simulink model "gm_inc_enc_v25_vnl"  (R2022a)
settings: Solver=FixedStepDiscrete  StartTime=0.0  StopTime=SimulationsDauer  RelTol=1e-3
undefined symbols (not defined in the file or in its folder): DiscIntNeverNeededParam, f_ISR, IncPerTurn, inital_zero_speed_timeout, n_max, OmegaPerOverSampl, Periode, Phase_Delay_A, Phase_Delay_B, PolePair, QuadratureFactor, reciprocal_iterations, T_fpga, T_mech
libraries: simulink x19, hdlsllib x11, hdlmdlgenlib x4, dspsrcs4 x3, dspswit3 x2, spsEdgeDetectorLib x2, simulink_extras x1
(part 1 of 4)
settings Model: Creator=Wendel_ELSYS  LastModifiedBy=ga92wum
settings SolverCC: ConcurrentTasks=on  AlgebraicLoopSolver=TrustRegion  MinimalZcImpactIntegration=on
settings DataIOCC: LimitDataPoints=on  SaveFormat=Array
settings OptimizationCC: BlockReduction=off  ConditionallyExecuteInputs=off  DefaultParameterBehavior=Inlined  InheritOutputTypeSmallerThanSingle=on  LifeSpan=inf
settings DebuggingCC: ReadBeforeWriteMsg=DisableAll  WriteAfterWriteMsg=DisableAll  WriteAfterReadMsg=DisableAll  AlgebraicLoopMsg=error  InheritedTsInSrcMsg=none  SingleTaskRateTransMsg=error  ParameterOverflowMsg=none  UnconnectedInputMsg=warning  UnconnectedOutputMsg=warning  UnconnectedLineMsg=warning  SFUnexpectedBacktrackingDiag=warning  SFNoUnconditionalDefaultTransitionDiag=warning  SFExecutionAtInitializationDiag=none  SFMachineParentedDataDiag=warning  ArithmeticOperatorsInVariantConditions=warning
settings HardwareCC: ProdBitPerPointer=32  ProdBitPerSizeT=32  ProdBitPerPtrDiffT=32  ProdLargestAtomicFloat=None  ProdIntDivRoundTo=Undefined  ProdEndianess=Unspecified  ProdWordSize=32  ProdHWDeviceType=ASIC/FPGA->ASIC/FPGA  ProdEqTarget=off
settings ModelReferenceCC: UpdateModelReferenceTargets=IfOutOfDate  PropagateSignalLabelsOutOfModel=off
settings SFSimCC: SFSimEcho=off  SimUseLocalCustomCode=off  CustomCodeUndefinedFunction=UseInterfaceOnly
settings RTWCC: RTWUseLocalCustomCode=off  DLArmComputeVersion=19.05
settings CodeAppCC: StateflowObjectComments=on
settings GRTTargetCC: TargetLangStandard=C89/C90 (ANSI)
settings ConfigComp: CovMetricSettings=dw  CovSaveCumulativeToWorkspaceVar=on  CovSaveSingleToWorkspaceVar=on  CovExternalEMLEnable=off

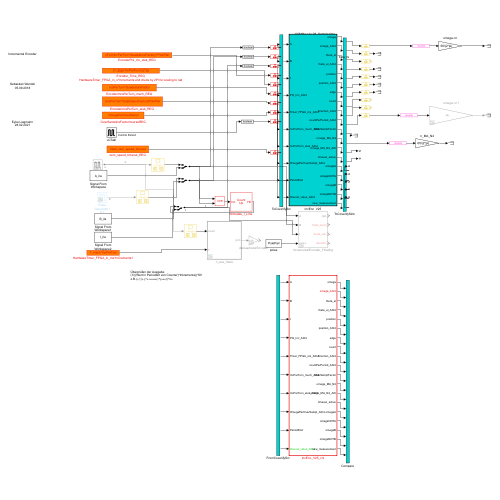
[thumbnail: Simulink's stored preview of the top-level diagram]
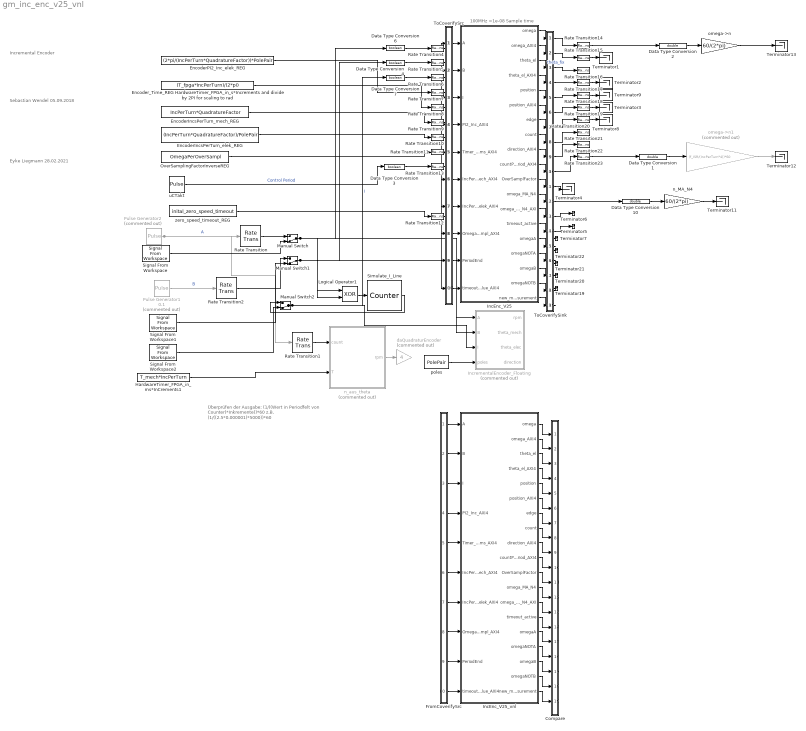
== system gm_inc_enc_v25_vnl ==
  note: 100MHz =1e-08 Sample time
  note: Überprüfen der Ausgabe:
      | (1/((Wert in Periodfelt von Counter)*Inkremente))*60
      | z.B. (1/((2.5*0.000001)*5000))*60
  note: Sebastian Wendel
      | 05.09.2018
  note: Incremental Encoder
  note: Eyke Liegmann
      | 28.02.2021
  Compare : Subsystem
      mask Display: disp('')
  Data Type Conversion1 : DataTypeConversion  OutDataTypeStr=double  SaturateOnIntegerOverflow=off  RndMeth=Floor
  Data Type Conversion10 : DataTypeConversion  OutDataTypeStr=double  SaturateOnIntegerOverflow=off  RndMeth=Floor
  Data Type Conversion2 : DataTypeConversion  OutDataTypeStr=double  SaturateOnIntegerOverflow=off  RndMeth=Floor
  Data Type Conversion{3..4,6..7} (4 alike) : DataTypeConversion  OutDataTypeStr=boolean  SaturateOnIntegerOverflow=off  RndMeth=Floor
  "EncoderIncsPerTurn_elek_REG " : Constant  Value=(IncPerTurn*QuadratureFactor)/PolePair  OutDataTypeStr=fixdt(0,16,0)  SampleTime=T_mech
  EncoderIncsPerTurn_mech_REG : Constant  Value=IncPerTurn*QuadratureFactor  OutDataTypeStr=fixdt(0,16,0)  SampleTime=T_mech
  EncoderPI2_Inc_elek_REG : Constant  Value=(2*pi/(IncPerTurn*QuadratureFactor))*PolePair  OutDataTypeStr=fixdt(0,24,24)  SampleTime=T_mech
  Encoder_Time_REG HardwareTimer_FPGA_in_s*Increments and divide by 2PI for scaling to rad : Constant  Value=(T_fpga*IncPerTurn)/(2*pi)  OutDataTypeStr=fixdt(0,32,32)  SampleTime=T_mech
  FromCoverifySrc : Subsystem
      mask Display: disp('')
  HardwareTimer_FPGA_in_ms*InCrements1 : Constant  Value=T_mech*IncPerTurn  OutDataTypeStr=double  SampleTime=T_mech
  IncEnc_V25 : Subsystem  TreatAsAtomicUnit=on
  IncEnc_V25_vnl : Subsystem  TreatAsAtomicUnit=on
  IncrementalEncoder_Floating : Subsystem  Commented=on
  Logical Operator1 : Logic  Operator=XOR  AllPortsSameDT=off  OutDataTypeStr=boolean
  Manual Switch : ManualSwitch  CurrentSetting=0
  Manual Switch1 : ManualSwitch  CurrentSetting=0
  Manual Switch2 : ManualSwitch  CurrentSetting=0
  OverSamplingFactorInverseREG : Constant  Value=OmegaPerOverSampl  OutDataTypeStr=fixdt(1,24,11)  SampleTime=T_mech
  Pulse Generator1 0.1 : DiscretePulseGenerator  Commented=on  PulseType=Time based  Period=Periode  PulseWidth=50  PhaseDelay=Phase_Delay_B  SampleTime=T_mech  VectorParams1D=off
  Pulse Generator2 : DiscretePulseGenerator  Commented=on  PulseType=Time based  Period=Periode  PulseWidth=50  PhaseDelay=Phase_Delay_A  SampleTime=T_mech  VectorParams1D=off
  Rate Transition{,1..2,14..23} (13 alike) : RateTransition  Deterministic=off  OutPortSampleTime=T_mech
  Rate Transition{4..13} (10 alike) : RateTransition  Deterministic=off  OutPortSampleTime=T_fpga
  Signal From Workspace : dspsrcs4/Signal From Workspace  X=A_ila  Ts=T_mech  nsamps=1  OutputAfterFinalValue=Setting to zero  ignoreOrWarnInputAndFrameLengths=off  OutputFrames=off
  Signal From Workspace1 : dspsrcs4/Signal From Workspace  X=B_ila  Ts=T_mech  nsamps=1  OutputAfterFinalValue=Setting to zero  ignoreOrWarnInputAndFrameLengths=off  OutputFrames=off
  Signal From Workspace2 : dspsrcs4/Signal From Workspace  X=I_ila  Ts=T_mech  nsamps=1  OutputAfterFinalValue=Setting to zero  ignoreOrWarnInputAndFrameLengths=off  OutputFrames=off
  Simulate_I_Line : dspswit3/Counter  Direction=Up  CountEvent=Either edge  CounterSize=User defined  MaxCount=IncPerTurn*4  InitialCount=0  Output=Hit  HitValue=IncPerTurn*4  ResetInput=off  SamplesPerFrame=1  Ts=1  CntDtype=double  HitDtype=Boolean
  Terminator{1..9,11..13,19..22} (16 alike) : Terminator
  ToCoverifySink : Subsystem
      mask Display: disp('')
  ToCoverifySrc : Subsystem
      mask Display: disp('')
  "daQuadraturEncoder " : Gain  Commented=on  Gain=4
  n_MA_N4 : Gain  Gain=60/(2*pi)  OutDataTypeStr=double
  n_aus_theta : Subsystem  Commented=on  TreatAsAtomicUnit=on
  omega->n : Gain  Gain=60/(2*pi)  OutDataTypeStr=double
  omega->n1 : Gain  Commented=on  Gain=(f_ISR/(IncPerTurn*4))*60  OutDataTypeStr=double
  poles : Constant  Value=PolePair  OutDataTypeStr=uint8  SampleTime=T_mech
  uCTakt : DiscretePulseGenerator  PulseType=Time based  Period=1/f_ISR  PulseWidth=f_ISR*T_fpga *100  SampleTime=T_mech  VectorParams1D=off
  zero_speed_timeout_REG : Constant  Value=inital_zero_speed_timeout  OutDataTypeStr=uint32  SampleTime=T_mech
  wires:
  Pulse Generator1 0.1/1 -> Rate Transition2/1  "B"
  Manual Switch1/1 -> Logical Operator1/2, Data Type Conversion4/1, IncrementalEncoder_Floating/2(B)
  Manual Switch2/1 -> Data Type Conversion7/1, IncrementalEncoder_Floating/3(I)  "I"
  Logical Operator1/1 -> Simulate_I_Line/1
  Manual Switch/1 -> Data Type Conversion6/1, IncrementalEncoder_Floating/1(A), Logical Operator1/1
  Data Type Conversion6/1 -> Rate Transition4/1
  Data Type Conversion4/1 -> Rate Transition5/1
  Data Type Conversion7/1 -> Rate Transition6/1
  poles/1 -> IncrementalEncoder_Floating/4(poles)
  EncoderPI2_Inc_elek_REG/1 -> Rate Transition7/1
  Encoder_Time_REG HardwareTimer_FPGA_in_s*Increments and divide by 2PI for scaling to rad/1 -> Rate Transition8/1
  EncoderIncsPerTurn_mech_REG/1 -> Rate Transition9/1
  "EncoderIncsPerTurn_elek_REG "/1 -> Rate Transition10/1
  omega->n/1 -> Terminator13/1
  Data Type Conversion2/1 -> omega->n/1
  HardwareTimer_FPGA_in_ms*InCrements1/1 -> n_aus_theta/2(T)
  Rate Transition1/1 -> n_aus_theta/1(count)
  n_aus_theta/1(rpm) -> "daQuadraturEncoder "/1
  Pulse Generator2/1 -> Rate Transition/1, Rate Transition1/1  "A"
  OverSamplingFactorInverseREG/1 -> Rate Transition11/1
  Rate Transition2/1 -> Manual Switch1/1
  Rate Transition/1 -> Manual Switch/1
  uCTakt/1 -> Data Type Conversion3/1  "Control Period"
  Data Type Conversion1/1 -> omega->n1/1
  Data Type Conversion3/1 -> Rate Transition13/1
  Rate Transition14/1 -> Data Type Conversion2/1
  Rate Transition15/1 -> Terminator1/1
  Rate Transition17/1 -> Terminator2/1
  Rate Transition19/1 -> Terminator3/1
  Rate Transition23/1 -> Data Type Conversion1/1
  Signal From Workspace/1 -> Manual Switch/2
  Signal From Workspace1/1 -> Manual Switch1/2
  Signal From Workspace2/1 -> Manual Switch2/2
  Simulate_I_Line/1 -> Manual Switch2/1
  Data Type Conversion10/1 -> n_MA_N4/1
  zero_speed_timeout_REG/1 -> Rate Transition12/1
  Rate Transition20/1 -> Terminator8/1
  Rate Transition18/1 -> Terminator9/1
  n_MA_N4/1 -> Terminator11/1
  omega->n1/1 -> Terminator12/1
  ToCoverifySrc/1(out1) -> IncEnc_V25/1(A)
  ToCoverifySrc/2(out2) -> IncEnc_V25/2(B)
  ToCoverifySrc/3(out3) -> IncEnc_V25/3(I)
  ToCoverifySrc/4(out4) -> IncEnc_V25/4(PI2_Inc_AXI4)
  ToCoverifySrc/5(out5) -> IncEnc_V25/5(Timer_FPGA_ms_AXI4)
  ToCoverifySrc/6(out6) -> IncEnc_V25/6(IncPerTurn_mech_AXI4)
  ToCoverifySrc/7(out7) -> IncEnc_V25/7(IncPerTurn_elek_AXI4)
  ToCoverifySrc/8(out8) -> IncEnc_V25/8(OmegaPerOverSampl_AXI4)
  ToCoverifySrc/9(out9) -> IncEnc_V25/9(PeriodEnd)
  ToCoverifySrc/10(out10) -> IncEnc_V25/10(timeout_value_AXI4)
  IncEnc_V25/1(omega) -> ToCoverifySink/1(in1)
  IncEnc_V25/2(omega_AXI4) -> ToCoverifySink/2(in2)
  IncEnc_V25/3(theta_el) -> ToCoverifySink/3(in3)  "theta_fix"
  IncEnc_V25/4(theta_el_AXI4) -> ToCoverifySink/4(in4)
  IncEnc_V25/5(position) -> ToCoverifySink/5(in5)
  IncEnc_V25/6(position_AXI4) -> ToCoverifySink/6(in6)
  IncEnc_V25/7(edge) -> ToCoverifySink/7(in7)
  IncEnc_V25/8(count) -> ToCoverifySink/8(in8)
  IncEnc_V25/9(direction_AXI4) -> ToCoverifySink/9(in9)
  IncEnc_V25/10(countPerPeriod_AXI4) -> ToCoverifySink/10(in10)
  IncEnc_V25/11(OverSamplFactor) -> ToCoverifySink/11(in11)
  IncEnc_V25/12(omega_MA_N4) -> ToCoverifySink/12(in12)
  IncEnc_V25/13(omega_MA_N4_AXI) -> ToCoverifySink/13(in13)
  IncEnc_V25/14(timeout_active) -> ToCoverifySink/14(in14)
  IncEnc_V25/15(omegaA) -> ToCoverifySink/15(in15)
  IncEnc_V25/16(omegaNOTA) -> ToCoverifySink/16(in16)
  IncEnc_V25/17(omegaB) -> ToCoverifySink/17(in17)
  IncEnc_V25/18(omegaNOTB) -> ToCoverifySink/18(in18)
  IncEnc_V25/19(new_measurement) -> ToCoverifySink/19(in19)
  Rate Transition4/1 -> ToCoverifySrc/1(in1)
  Rate Transition5/1 -> ToCoverifySrc/2(in2)
  Rate Transition6/1 -> ToCoverifySrc/3(in3)
  Rate Transition7/1 -> ToCoverifySrc/4(in4)
  Rate Transition8/1 -> ToCoverifySrc/5(in5)
  Rate Transition9/1 -> ToCoverifySrc/6(in6)
  Rate Transition10/1 -> ToCoverifySrc/7(in7)
  Rate Transition11/1 -> ToCoverifySrc/8(in8)
  Rate Transition13/1 -> ToCoverifySrc/9(in9)
  Rate Transition12/1 -> ToCoverifySrc/10(in10)
  ToCoverifySink/1(out1) -> Rate Transition14/1
  ToCoverifySink/2(out2) -> Rate Transition15/1
  ToCoverifySink/3(out3) -> Rate Transition16/1
  ToCoverifySink/4(out4) -> Rate Transition17/1
  ToCoverifySink/5(out5) -> Rate Transition18/1
  ToCoverifySink/6(out6) -> Rate Transition19/1
  ToCoverifySink/7(out7) -> Rate Transition20/1
  ToCoverifySink/8(out8) -> Rate Transition21/1
  ToCoverifySink/9(out9) -> Rate Transition22/1
  ToCoverifySink/10(out10) -> Rate Transition23/1
  ToCoverifySink/11(out11) -> Terminator4/1
  ToCoverifySink/12(out12) -> Data Type Conversion10/1
  ToCoverifySink/13(out13) -> Terminator6/1
  ToCoverifySink/14(out14) -> Terminator5/1
  ToCoverifySink/15(out15) -> Terminator7/1
  ToCoverifySink/16(out16) -> Terminator22/1
  ToCoverifySink/17(out17) -> Terminator21/1
  ToCoverifySink/18(out18) -> Terminator20/1
  ToCoverifySink/19(out19) -> Terminator19/1
  FromCoverifySrc/1(out1) -> IncEnc_V25_vnl/1(A)
  FromCoverifySrc/2(out2) -> IncEnc_V25_vnl/2(B)
  FromCoverifySrc/3(out3) -> IncEnc_V25_vnl/3(I)
  FromCoverifySrc/4(out4) -> IncEnc_V25_vnl/4(PI2_Inc_AXI4)
  FromCoverifySrc/5(out5) -> IncEnc_V25_vnl/5(Timer_FPGA_ms_AXI4)
  FromCoverifySrc/6(out6) -> IncEnc_V25_vnl/6(IncPerTurn_mech_AXI4)
  FromCoverifySrc/7(out7) -> IncEnc_V25_vnl/7(IncPerTurn_elek_AXI4)
  FromCoverifySrc/8(out8) -> IncEnc_V25_vnl/8(OmegaPerOverSampl_AXI4)
  FromCoverifySrc/9(out9) -> IncEnc_V25_vnl/9(PeriodEnd)
  FromCoverifySrc/10(out10) -> IncEnc_V25_vnl/10(timeout_value_AXI4)
  IncEnc_V25_vnl/1(omega) -> Compare/1(in1)
  IncEnc_V25_vnl/2(omega_AXI4) -> Compare/2(in2)
  IncEnc_V25_vnl/3(theta_el) -> Compare/3(in3)
  IncEnc_V25_vnl/4(theta_el_AXI4) -> Compare/4(in4)
  IncEnc_V25_vnl/5(position) -> Compare/5(in5)
  IncEnc_V25_vnl/6(position_AXI4) -> Compare/6(in6)
  IncEnc_V25_vnl/7(edge) -> Compare/7(in7)
  IncEnc_V25_vnl/8(count) -> Compare/8(in8)
  IncEnc_V25_vnl/9(direction_AXI4) -> Compare/9(in9)
  IncEnc_V25_vnl/10(countPerPeriod_AXI4) -> Compare/10(in10)
  IncEnc_V25_vnl/11(OverSamplFactor) -> Compare/11(in11)
  IncEnc_V25_vnl/12(omega_MA_N4) -> Compare/12(in12)
  IncEnc_V25_vnl/13(omega_MA_N4_AXI) -> Compare/13(in13)
  IncEnc_V25_vnl/14(timeout_active) -> Compare/14(in14)
  IncEnc_V25_vnl/15(omegaA) -> Compare/15(in15)
  IncEnc_V25_vnl/16(omegaNOTA) -> Compare/16(in16)
  IncEnc_V25_vnl/17(omegaB) -> Compare/17(in17)
  IncEnc_V25_vnl/18(omegaNOTB) -> Compare/18(in18)
  IncEnc_V25_vnl/19(new_measurement) -> Compare/19(in19)

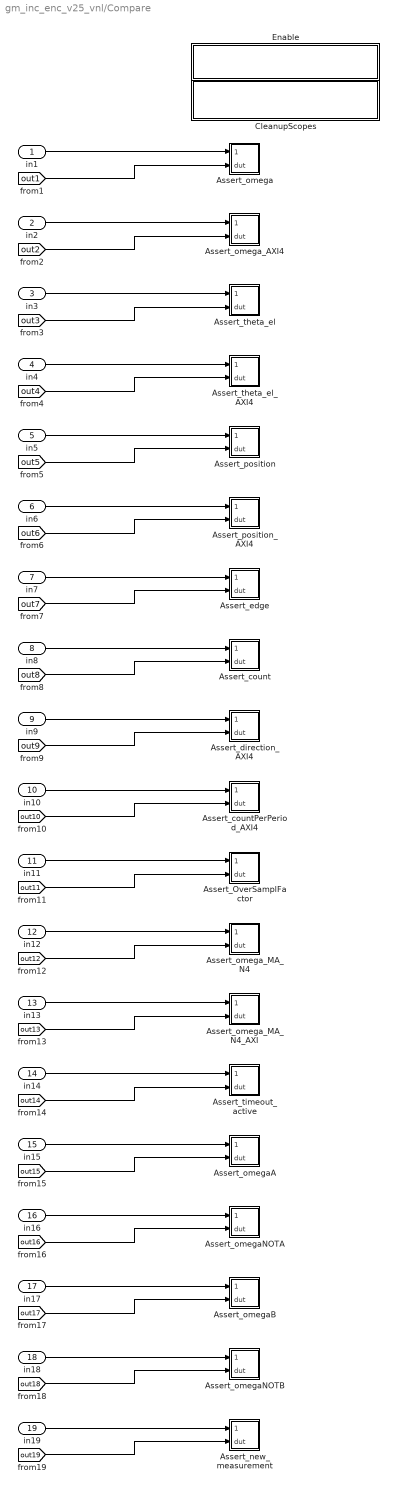
== system gm_inc_enc_v25_vnl/Compare ==
  in1 : Inport
  in2 : Inport  Port=2
  in3 : Inport  Port=3
  in4 : Inport  Port=4
  in5 : Inport  Port=5
  in6 : Inport  Port=6
  in7 : Inport  Port=7
  in8 : Inport  Port=8
  in9 : Inport  Port=9
  in10 : Inport  Port=10
  in11 : Inport  Port=11
  in12 : Inport  Port=12
  in13 : Inport  Port=13
  in14 : Inport  Port=14
  in15 : Inport  Port=15
  in16 : Inport  Port=16
  in17 : Inport  Port=17
  in18 : Inport  Port=18
  in19 : Inport  Port=19
  Assert_OverSamplFactor : Subsystem
  Assert_count : Subsystem
  Assert_countPerPeriod_AXI4 : Subsystem
  Assert_direction_AXI4 : Subsystem
  Assert_edge : Subsystem
  Assert_new_measurement : Subsystem
  Assert_omega : Subsystem
  Assert_omegaA : Subsystem
  Assert_omegaB : Subsystem
  Assert_omegaNOTA : Subsystem
  Assert_omegaNOTB : Subsystem
  Assert_omega_AXI4 : Subsystem
  Assert_omega_MA_N4 : Subsystem
  Assert_omega_MA_N4_AXI : Subsystem
  Assert_position : Subsystem
  Assert_position_AXI4 : Subsystem
  Assert_theta_el : Subsystem
  Assert_theta_el_AXI4 : Subsystem
  Assert_timeout_active : Subsystem
  CleanupScopes : Subsystem
      settings: OpenFcn=|
      | blkName = gcb; %self block
      | idx = regexp(blkName, '/CleanupScopes$', 'once');
      | blkParent = blkName(1:idx-1);
      | blks=find_system(blkParent, 'LookUnderMasks', 'all','blocktype', 'Scope');
      | for itr = 1:length(blks)
      | 	 hScopeCfg = get_param(blks{itr},'ScopeConfiguration');
      | 	 hScopeCfg.Visible = ~ hScopeCfg.Visible;
      | end
      | drawnow;
      mask Display: fprintf(message('hdlcoder:cosim:vnl_dblclick').getString());
  Enable : Subsystem
      settings: OpenFcn=|
      | blkName = gcb;
      | idx = regexp(blkName, '/Enable$', 'once');
      | blkParent = blkName(1:idx-1);
      | blks=find_system(blkParent, 'LookUnderMasks', 'all','blocktype', 'Assertion');
      | e = get_param(blks{1}, 'Enabled');
      | if strcmp(e, 'on'), f= 'off';, else, f = 'on';, end
      | for ii=1:length(blks), set_param(blks{ii}, 'Enabled', f);, end
      | set_param(gcb, 'MaskDisplay',['fprintf(message(''hdlcoder:cosim:vnl_dblclick_assertions'',','''',upper(e),'''',').getString())']);
      mask Display: fprintf(message('hdlcoder:cosim:vnl_dblclick_assertions','OFF').getString());
  wires:
  in1/1 -> Assert_omega/1(cosim)
  [out1] -> Assert_omega/2(dut)
  in2/1 -> Assert_omega_AXI4/1(cosim)
  [out2] -> Assert_omega_AXI4/2(dut)
  in3/1 -> Assert_theta_el/1(cosim)
  [out3] -> Assert_theta_el/2(dut)
  in4/1 -> Assert_theta_el_AXI4/1(cosim)
  [out4] -> Assert_theta_el_AXI4/2(dut)
  in5/1 -> Assert_position/1(cosim)
  [out5] -> Assert_position/2(dut)
  in6/1 -> Assert_position_AXI4/1(cosim)
  [out6] -> Assert_position_AXI4/2(dut)
  in7/1 -> Assert_edge/1(cosim)
  [out7] -> Assert_edge/2(dut)
  in8/1 -> Assert_count/1(cosim)
  [out8] -> Assert_count/2(dut)
  in9/1 -> Assert_direction_AXI4/1(cosim)
  [out9] -> Assert_direction_AXI4/2(dut)
  in10/1 -> Assert_countPerPeriod_AXI4/1(cosim)
  [out10] -> Assert_countPerPeriod_AXI4/2(dut)
  in11/1 -> Assert_OverSamplFactor/1(cosim)
  [out11] -> Assert_OverSamplFactor/2(dut)
  in12/1 -> Assert_omega_MA_N4/1(cosim)
  [out12] -> Assert_omega_MA_N4/2(dut)
  in13/1 -> Assert_omega_MA_N4_AXI/1(cosim)
  [out13] -> Assert_omega_MA_N4_AXI/2(dut)
  in14/1 -> Assert_timeout_active/1(cosim)
  [out14] -> Assert_timeout_active/2(dut)
  in15/1 -> Assert_omegaA/1(cosim)
  [out15] -> Assert_omegaA/2(dut)
  in16/1 -> Assert_omegaNOTA/1(cosim)
  [out16] -> Assert_omegaNOTA/2(dut)
  in17/1 -> Assert_omegaB/1(cosim)
  [out17] -> Assert_omegaB/2(dut)
  in18/1 -> Assert_omegaNOTB/1(cosim)
  [out18] -> Assert_omegaNOTB/2(dut)
  in19/1 -> Assert_new_measurement/1(cosim)
  [out19] -> Assert_new_measurement/2(dut)

== system gm_inc_enc_v25_vnl/FromCoverifySrc ==
  out1 : Outport
  out2 : Outport  Port=2
  out3 : Outport  Port=3
  out4 : Outport  Port=4
  out5 : Outport  Port=5
  out6 : Outport  Port=6
  out7 : Outport  Port=7
  out8 : Outport  Port=8
  out9 : Outport  Port=9
  out10 : Outport  Port=10
  wires:
  [in1] -> out1/1
  [in2] -> out2/1
  [in3] -> out3/1
  [in4] -> out4/1
  [in5] -> out5/1
  [in6] -> out6/1
  [in7] -> out7/1
  [in8] -> out8/1
  [in9] -> out9/1
  [in10] -> out10/1

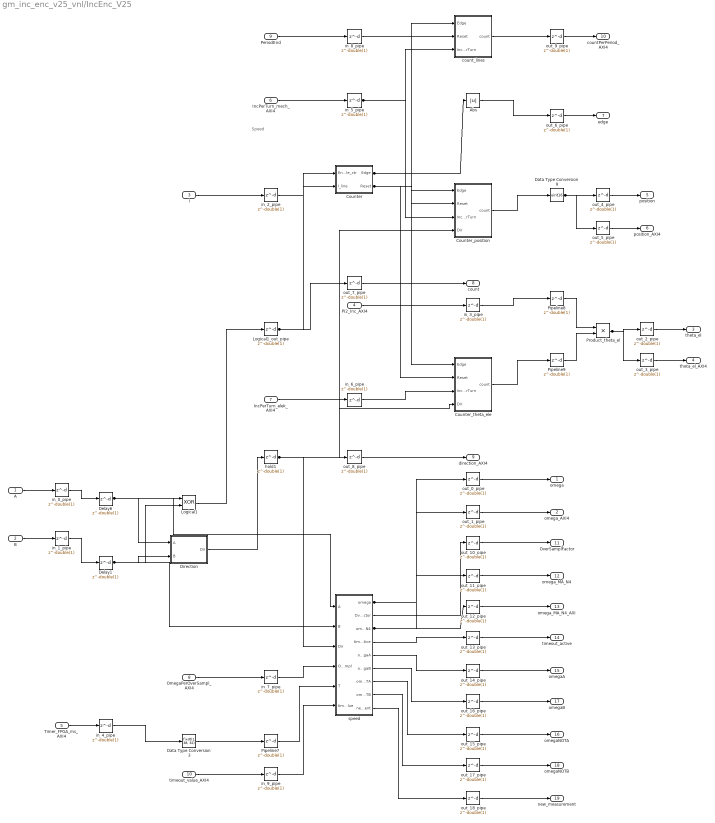
== system gm_inc_enc_v25_vnl/IncEnc_V25 ==
  note: Speed
  A : Inport  OutDataTypeStr=boolean  PortDimensions=1  SampleTime=1e-08
  B : Inport  Port=2  OutDataTypeStr=boolean  PortDimensions=1  SampleTime=1e-08
  I : Inport  Port=3  OutDataTypeStr=boolean  PortDimensions=1  SampleTime=1e-08
  PI2_Inc_AXI4 : Inport  Port=4  OutDataTypeStr=fixdt(0, 24, 24)  PortDimensions=1  SampleTime=1e-08
  Timer_FPGA_ms_AXI4 : Inport  Port=5  OutDataTypeStr=fixdt(0, 32, 32)  PortDimensions=1  SampleTime=1e-08
  IncPerTurn_mech_AXI4 : Inport  Port=6  OutDataTypeStr=uint16  PortDimensions=1  SampleTime=1e-08
  IncPerTurn_elek_AXI4 : Inport  Port=7  OutDataTypeStr=uint16  PortDimensions=1  SampleTime=1e-08
  OmegaPerOverSampl_AXI4 : Inport  Port=8  OutDataTypeStr=fixdt(1, 24, 11)  PortDimensions=1  SampleTime=1e-08
  PeriodEnd : Inport  Port=9  OutDataTypeStr=boolean  PortDimensions=1  SampleTime=1e-08
  timeout_value_AXI4 : Inport  Port=10  OutDataTypeStr=uint32  PortDimensions=1  SampleTime=1e-08
  Abs : Abs  SampleTime=1e-08  OutDataTypeStr=fixdt(0, 1, 0)  RndMeth=Simplest  SaturateOnIntegerOverflow=off
  Counter : Subsystem
  Counter_position : Subsystem
  Counter_theta_ele : Subsystem
  Data Type Conversion3 : DataTypeConversion  OutDataTypeStr=fixdt(1, 38, 32)  SampleTime=1e-08  SaturateOnIntegerOverflow=off  RndMeth=Floor
  Data Type Conversion9 : DataTypeConversion  OutDataTypeStr=uint16  SampleTime=1e-08  SaturateOnIntegerOverflow=off  RndMeth=Floor
  Delay1 : Delay  DelayLength=double(1)  InitialCondition=0  SampleTime=1e-08
  Delay6 : Delay  DelayLength=double(1)  InitialCondition=0  SampleTime=1e-08
  Direction : Subsystem
  Logical1 : Logic  Operator=XOR  AllPortsSameDT=off  OutDataTypeStr=boolean  SampleTime=1e-08
  Logical1_out_pipe : Delay  DelayLength=double(1)  InitialCondition=0  SampleTime=1e-08
  Pipeline7 : Delay  DelayLength=double(1)  InitialCondition=0  SampleTime=1e-08
  Pipeline8 : Delay  DelayLength=double(1)  InitialCondition=0  SampleTime=1e-08
  Pipeline9 : Delay  DelayLength=double(1)  InitialCondition=0  SampleTime=1e-08
  Product_theta_el : Product  Inputs=**  OutDataTypeStr=fixdt(1, 24, 20)  SampleTime=1e-08
  count_lines : Subsystem
  hold1 : Delay  DelayLength=double(1)  InitialCondition=0  SampleTime=1e-08
  in_0_pipe : Delay  DelayLength=double(1)  InitialCondition=0  SampleTime=1e-08
  in_1_pipe : Delay  DelayLength=double(1)  InitialCondition=0  SampleTime=1e-08
  in_2_pipe : Delay  DelayLength=double(1)  InitialCondition=0  SampleTime=1e-08
  in_3_pipe : Delay  DelayLength=double(1)  InitialCondition=0  SampleTime=1e-08
  in_4_pipe : Delay  DelayLength=double(1)  InitialCondition=0  SampleTime=1e-08
  in_5_pipe : Delay  DelayLength=double(1)  InitialCondition=0  SampleTime=1e-08
  in_6_pipe : Delay  DelayLength=double(1)  InitialCondition=0  SampleTime=1e-08
  in_7_pipe : Delay  DelayLength=double(1)  InitialCondition=0  SampleTime=1e-08
  in_8_pipe : Delay  DelayLength=double(1)  InitialCondition=0  SampleTime=1e-08
  in_9_pipe : Delay  DelayLength=double(1)  InitialCondition=0  SampleTime=1e-08
  out_0_pipe : Delay  DelayLength=double(1)  InitialCondition=0  SampleTime=1e-08
  out_10_pipe : Delay  DelayLength=double(1)  InitialCondition=0  SampleTime=1e-08
  out_11_pipe : Delay  DelayLength=double(1)  InitialCondition=0  SampleTime=1e-08
  out_12_pipe : Delay  DelayLength=double(1)  InitialCondition=0  SampleTime=1e-08
  out_13_pipe : Delay  DelayLength=double(1)  InitialCondition=0  SampleTime=1e-08
  out_14_pipe : Delay  DelayLength=double(1)  InitialCondition=0  SampleTime=1e-08
  out_15_pipe : Delay  DelayLength=double(1)  InitialCondition=0  SampleTime=1e-08
  out_16_pipe : Delay  DelayLength=double(1)  InitialCondition=0  SampleTime=1e-08
  out_17_pipe : Delay  DelayLength=double(1)  InitialCondition=0  SampleTime=1e-08
  out_18_pipe : Delay  DelayLength=double(1)  InitialCondition=0  SampleTime=1e-08
  out_1_pipe : Delay  DelayLength=double(1)  InitialCondition=0  SampleTime=1e-08
  out_2_pipe : Delay  DelayLength=double(1)  InitialCondition=0  SampleTime=1e-08
  out_3_pipe : Delay  DelayLength=double(1)  InitialCondition=0  SampleTime=1e-08
  out_4_pipe : Delay  DelayLength=double(1)  InitialCondition=0  SampleTime=1e-08
  out_5_pipe : Delay  DelayLength=double(1)  InitialCondition=0  SampleTime=1e-08
  out_6_pipe : Delay  DelayLength=double(1)  InitialCondition=0  SampleTime=1e-08
  out_7_pipe : Delay  DelayLength=double(1)  InitialCondition=0  SampleTime=1e-08
  out_8_pipe : Delay  DelayLength=double(1)  InitialCondition=0  SampleTime=1e-08
  out_9_pipe : Delay  DelayLength=double(1)  InitialCondition=0  SampleTime=1e-08
  speed : Subsystem
  omega : Outport  SampleTime=1e-08  VectorParamsAs1DForOutWhenUnconnected=off
  omega_AXI4 : Outport  Port=2  SampleTime=1e-08  VectorParamsAs1DForOutWhenUnconnected=off
  theta_el : Outport  Port=3  SampleTime=1e-08  VectorParamsAs1DForOutWhenUnconnected=off
  theta_el_AXI4 : Outport  Port=4  SampleTime=1e-08  VectorParamsAs1DForOutWhenUnconnected=off
  position : Outport  Port=5  SampleTime=1e-08  VectorParamsAs1DForOutWhenUnconnected=off
  position_AXI4 : Outport  Port=6  SampleTime=1e-08  VectorParamsAs1DForOutWhenUnconnected=off
  edge : Outport  Port=7  SampleTime=1e-08  VectorParamsAs1DForOutWhenUnconnected=off
  count : Outport  Port=8  SampleTime=1e-08  VectorParamsAs1DForOutWhenUnconnected=off
  direction_AXI4 : Outport  Port=9  SampleTime=1e-08  VectorParamsAs1DForOutWhenUnconnected=off
  countPerPeriod_AXI4 : Outport  Port=10  SampleTime=1e-08  VectorParamsAs1DForOutWhenUnconnected=off
  OverSamplFactor : Outport  Port=11  SampleTime=1e-08  VectorParamsAs1DForOutWhenUnconnected=off
  omega_MA_N4 : Outport  Port=12  SampleTime=1e-08  VectorParamsAs1DForOutWhenUnconnected=off
  omega_MA_N4_AXI : Outport  Port=13  SampleTime=1e-08  VectorParamsAs1DForOutWhenUnconnected=off
  timeout_active : Outport  Port=14  OutDataTypeStr=boolean  SampleTime=1e-08  VectorParamsAs1DForOutWhenUnconnected=off
  omegaA : Outport  Port=15  SampleTime=1e-08  VectorParamsAs1DForOutWhenUnconnected=off
  omegaNOTA : Outport  Port=16  SampleTime=1e-08  VectorParamsAs1DForOutWhenUnconnected=off
  omegaB : Outport  Port=17  SampleTime=1e-08  VectorParamsAs1DForOutWhenUnconnected=off
  omegaNOTB : Outport  Port=18  SampleTime=1e-08  VectorParamsAs1DForOutWhenUnconnected=off
  new_measurement : Outport  Port=19  OutDataTypeStr=boolean  SampleTime=1e-08  VectorParamsAs1DForOutWhenUnconnected=off
  wires:
  timeout_value_AXI4/1 -> in_9_pipe/1
  PeriodEnd/1 -> in_8_pipe/1
  OmegaPerOverSampl_AXI4/1 -> in_7_pipe/1
  IncPerTurn_elek_AXI4/1 -> in_6_pipe/1
  IncPerTurn_mech_AXI4/1 -> in_5_pipe/1
  Timer_FPGA_ms_AXI4/1 -> in_4_pipe/1
  PI2_Inc_AXI4/1 -> in_3_pipe/1
  I/1 -> in_2_pipe/1
  B/1 -> in_1_pipe/1
  A/1 -> in_0_pipe/1
  Logical1/1 -> Logical1_out_pipe/1
  out_18_pipe/1 -> new_measurement/1
  out_17_pipe/1 -> omegaNOTB/1
  out_16_pipe/1 -> omegaB/1
  out_15_pipe/1 -> omegaNOTA/1
  out_14_pipe/1 -> omegaA/1
  out_13_pipe/1 -> timeout_active/1
  out_12_pipe/1 -> omega_MA_N4_AXI/1
  out_11_pipe/1 -> omega_MA_N4/1
  out_10_pipe/1 -> OverSamplFactor/1
  out_9_pipe/1 -> countPerPeriod_AXI4/1
  out_8_pipe/1 -> direction_AXI4/1
  out_7_pipe/1 -> count/1
  out_6_pipe/1 -> edge/1
  out_5_pipe/1 -> position_AXI4/1
  out_4_pipe/1 -> position/1
  out_3_pipe/1 -> theta_el_AXI4/1
  out_2_pipe/1 -> theta_el/1
  out_1_pipe/1 -> omega_AXI4/1
  out_0_pipe/1 -> omega/1
  speed/9(new_measurement) -> out_18_pipe/1
  speed/8(omegaNOTB) -> out_17_pipe/1
  speed/7(omegaNOTA) -> out_15_pipe/1
  speed/6(omegaB) -> out_16_pipe/1
  speed/5(omegaA) -> out_14_pipe/1
  speed/4(timeout_active) -> out_13_pipe/1
  speed/3(omega_MA_N4) -> out_11_pipe/1, out_12_pipe/1
  speed/2(OverSamplFactor) -> out_10_pipe/1
  speed/1(omega) -> out_0_pipe/1, out_1_pipe/1
  hold1/1 -> speed/3(Dir), Counter_position/4(Dir), Counter_theta_ele/4(Dir), out_8_pipe/1
  count_lines/1(count) -> out_9_pipe/1
  Product_theta_el/1 -> out_2_pipe/1, out_3_pipe/1
  Pipeline9/1 -> Product_theta_el/2
  Pipeline8/1 -> Product_theta_el/1
  Pipeline7/1 -> speed/5(T)
  Logical1_out_pipe/1 -> Counter/1(Enable_ctr), out_7_pipe/1
  Direction/1(Dir) -> hold1/1
  Delay6/1 -> Direction/1(A), speed/1(A), Logical1/1
  Delay1/1 -> Direction/2(B), speed/2(B), Logical1/2
  Data Type Conversion9/1 -> out_4_pipe/1, out_5_pipe/1
  Data Type Conversion3/1 -> Pipeline7/1
  Counter_theta_ele/1(count) -> Pipeline9/1
  Counter_position/1(count) -> Data Type Conversion9/1
  Counter/2(Reset) -> Counter_position/2(Reset), Counter_theta_ele/2(Reset)
  Counter/1(Edge) -> count_lines/1(Edge), Counter_position/1(Edge), Counter_theta_ele/1(Edge), Abs/1
  Abs/1 -> out_6_pipe/1
  in_9_pipe/1 -> speed/6(timeout_value)
  in_8_pipe/1 -> count_lines/2(Reset)
  in_7_pipe/1 -> speed/4(OmegaPerOverSampl)
  in_6_pipe/1 -> Counter_theta_ele/3(IncsPerTurn)
  in_5_pipe/1 -> Counter_position/3(IncsPerTurn), count_lines/3(IncsPerTurn)
  in_4_pipe/1 -> Data Type Conversion3/1
  in_3_pipe/1 -> Pipeline8/1
  in_2_pipe/1 -> Counter/2(I_line)
  in_1_pipe/1 -> Delay1/1
  in_0_pipe/1 -> Delay6/1

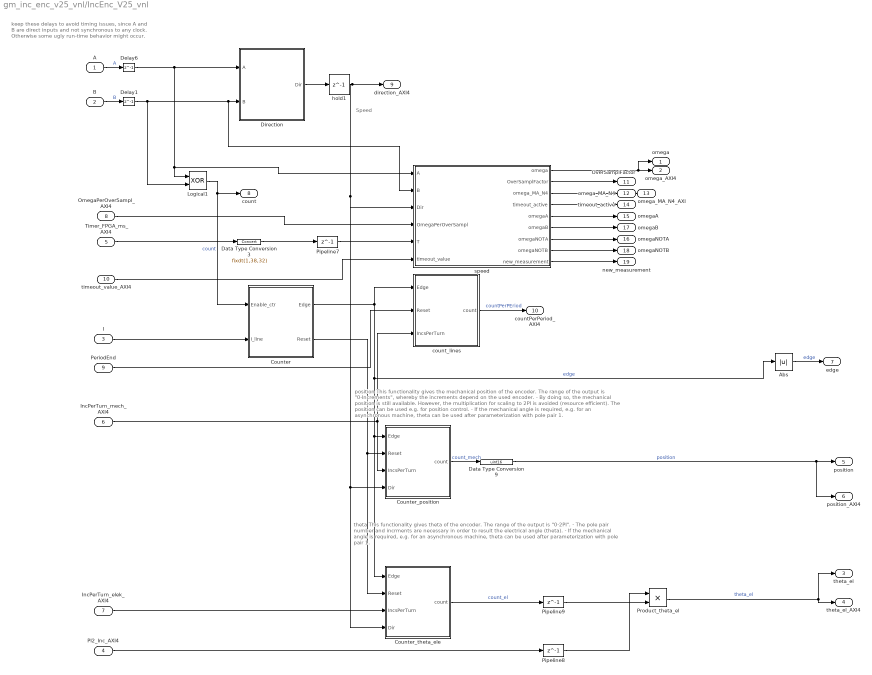
== system gm_inc_enc_v25_vnl/IncEnc_V25_vnl ==
  note: keep these delays to avoid timing issues,
      | since A and B are direct inputs and
      | not synchronous to any clock.
      | Otherwise some ugly run-time
      | behavior might occur.
  note: theta
      | This functionality gives theta of the encoder. The range of the output is "0-2PI".
      | - The pole pair number and incrments are necessary in order to result the electrical angle (theta).
      | - If the mechanical angle is required, e.g. for an asynchronous machine, theta can be used after parameterization with pole pair 1.
  note: position
      | This functionality gives the mechanical position of the encoder. The range of the output is "0-Increments", whereby the increments depend on the used encoder.
      | - By doing so, the mechanical position is still available. However, the multiplication for scaling to 2PI is avoided (resource efficient). The position can be used e.g. for position control.
      | - If the mechanical angle is required, e.g. for an asynchronous machine, theta can be used after parameterization with pole pair 1.
  note: Speed
  A : Inport
  B : Inport  Port=2
  I : Inport  Port=3
  PI2_Inc_AXI4 : Inport  Port=4
  Timer_FPGA_ms_AXI4 : Inport  Port=5
  IncPerTurn_mech_AXI4 : Inport  Port=6
  IncPerTurn_elek_AXI4 : Inport  Port=7
  OmegaPerOverSampl_AXI4 : Inport  Port=8
  PeriodEnd : Inport  Port=9
  timeout_value_AXI4 : Inport  Port=10  OutDataTypeStr=uint32
  Abs : Abs  OutDataTypeStr=fixdt(0,1,0)  RndMeth=Simplest  SaturateOnIntegerOverflow=off
  Counter : Subsystem  TreatAsAtomicUnit=on
  Counter_position : Subsystem  TreatAsAtomicUnit=on
  Counter_theta_ele : Subsystem  TreatAsAtomicUnit=on
  Data Type Conversion3 : DataTypeConversion  OutDataTypeStr=fixdt(1,38,32)  SaturateOnIntegerOverflow=off  RndMeth=Floor
  Data Type Conversion9 : DataTypeConversion  OutDataTypeStr=uint16  SaturateOnIntegerOverflow=off  RndMeth=Floor
  Delay1 : Delay  DelayLength=1  InitialCondition=0
  Delay6 : Delay  DelayLength=1  InitialCondition=0
  Direction : Subsystem  TreatAsAtomicUnit=on
  Logical1 : Logic  Operator=XOR  AllPortsSameDT=off  OutDataTypeStr=boolean
  Pipeline7 : Delay  DelayLength=1
  Pipeline8 : Delay  DelayLength=1
  Pipeline9 : Delay  DelayLength=1
  Product_theta_el : Product  OutMin=[0]  OutMax=[2*pi]  OutDataTypeStr=fixdt(1,24,20)
  count_lines : Subsystem  TreatAsAtomicUnit=on
  hold1 : Delay  DelayLength=1
  speed : Subsystem
  omega : Outport  VectorParamsAs1DForOutWhenUnconnected=off
  omega_AXI4 : Outport  Port=2  VectorParamsAs1DForOutWhenUnconnected=off
  theta_el : Outport  Port=3  VectorParamsAs1DForOutWhenUnconnected=off
  theta_el_AXI4 : Outport  Port=4  VectorParamsAs1DForOutWhenUnconnected=off
  position : Outport  Port=5  VectorParamsAs1DForOutWhenUnconnected=off
  position_AXI4 : Outport  Port=6  VectorParamsAs1DForOutWhenUnconnected=off
  edge : Outport  Port=7  VectorParamsAs1DForOutWhenUnconnected=off
  count : Outport  Port=8  VectorParamsAs1DForOutWhenUnconnected=off
  direction_AXI4 : Outport  Port=9  VectorParamsAs1DForOutWhenUnconnected=off
  countPerPeriod_AXI4 : Outport  Port=10  VectorParamsAs1DForOutWhenUnconnected=off
  OverSamplFactor : Outport  Port=11  VectorParamsAs1DForOutWhenUnconnected=off
  omega_MA_N4 : Outport  Port=12  VectorParamsAs1DForOutWhenUnconnected=off
  omega_MA_N4_AXI : Outport  Port=13  VectorParamsAs1DForOutWhenUnconnected=off
  timeout_active : Outport  Port=14  OutDataTypeStr=boolean  VectorParamsAs1DForOutWhenUnconnected=off
  omegaA : Outport  Port=15  VectorParamsAs1DForOutWhenUnconnected=off
  omegaNOTA : Outport  Port=16  VectorParamsAs1DForOutWhenUnconnected=off
  omegaB : Outport  Port=17  VectorParamsAs1DForOutWhenUnconnected=off
  omegaNOTB : Outport  Port=18  VectorParamsAs1DForOutWhenUnconnected=off
  new_measurement : Outport  Port=19  OutDataTypeStr=boolean  VectorParamsAs1DForOutWhenUnconnected=off
  wires:
  Delay1/1 -> Direction/2(B), speed/2(B), Logical1/2
  Delay6/1 -> Direction/1(A), speed/1(A), Logical1/1
  speed/9(new_measurement) -> new_measurement/1
  speed/8(omegaNOTB) -> omegaNOTB/1
  speed/6(omegaB) -> omegaB/1
  speed/7(omegaNOTA) -> omegaNOTA/1
  speed/5(omegaA) -> omegaA/1
  Pipeline9/1 -> Product_theta_el/2
  Pipeline8/1 -> Product_theta_el/1
  timeout_value_AXI4/1 -> speed/6(timeout_value)
  speed/4(timeout_active) -> timeout_active/1
  speed/3(omega_MA_N4) -> omega_MA_N4/1, omega_MA_N4_AXI/1
  speed/2(OverSamplFactor) -> OverSamplFactor/1
  speed/1(omega) -> omega_AXI4/1, omega/1
  Pipeline7/1 -> speed/5(T)
  OmegaPerOverSampl_AXI4/1 -> speed/4(OmegaPerOverSampl)
  Data Type Conversion3/1 -> Pipeline7/1
  Timer_FPGA_ms_AXI4/1 -> Data Type Conversion3/1
  IncPerTurn_mech_AXI4/1 -> Counter_position/3(IncsPerTurn), count_lines/3(IncsPerTurn)
  IncPerTurn_elek_AXI4/1 -> Counter_theta_ele/3(IncsPerTurn)
  PI2_Inc_AXI4/1 -> Pipeline8/1
  Abs/1 -> edge/1  "edge"
  count_lines/1(count) -> countPerPeriod_AXI4/1  "countPerPEriod"
  PeriodEnd/1 -> count_lines/2(Reset)
  Direction/1(Dir) -> hold1/1
  Counter/1(Edge) -> count_lines/1(Edge), Abs/1, Counter_position/1(Edge), Counter_theta_ele/1(Edge)  "edge"
  Counter/2(Reset) -> Counter_position/2(Reset), Counter_theta_ele/2(Reset)
  Product_theta_el/1 -> theta_el_AXI4/1, theta_el/1  "theta_el"
  Counter_theta_ele/1(count) -> Pipeline9/1  "count_el"
  Logical1/1 -> count/1, Counter/1(Enable_ctr)  "count"
  Data Type Conversion9/1 -> position/1, position_AXI4/1  "position"
  Counter_position/1(count) -> Data Type Conversion9/1  "count_mech"
  hold1/1 -> speed/3(Dir), Counter_position/4(Dir), Counter_theta_ele/4(Dir), direction_AXI4/1
  I/1 -> Counter/2(I_line)
  B/1 -> Delay1/1  "B"
  A/1 -> Delay6/1  "A"

== system gm_inc_enc_v25_vnl/IncrementalEncoder_Floating ==
  A : Inport
  B : Inport  Port=2
  I : Inport  Port=3
  poles : Inport  Port=4
  Add : Sum  Inputs=+-  OutDataTypeStr=fixdt(1,16,0)
  Counter3 : dspswit3/Counter  Direction=Up  CountEvent=Either edge  CounterSize=User defined  MaxCount=IncPerTurn*4  InitialCount=0  Output=Count  HitValue=32  ResetInput=on  SamplesPerFrame=1  Ts=1  CntDtype=double  HitDtype=Logical
  CutTheta_0_2PI : Subsystem
  Edge Detector2 : spsEdgeDetectorLib/Edge Detector  model=Rising  ic=0  Ts=-1
      settings: SourceProductBaseCode=PS
  Edge Detector3 : spsEdgeDetectorLib/Edge Detector  model=Rising  ic=0  Ts=-1
      settings: SourceProductBaseCode=PS
  Logical Operator1 : Logic  Operator=XOR  AllPortsSameDT=off  OutDataTypeStr=boolean
  Logical Operator3 : Logic  AllPortsSameDT=off  OutDataTypeStr=boolean
  Logical Operator4 : Logic  Operator=NOT  AllPortsSameDT=off  OutDataTypeStr=boolean
  Logical Operator5 : Logic  AllPortsSameDT=off  OutDataTypeStr=boolean
  Logical Operator6 : Logic  Operator=NOT  AllPortsSameDT=off  OutDataTypeStr=boolean
  Product : Product
  S-R Flip-Flop1 : simulink_extras/Flip Flops/S-R Flip-Flop  initial_condition=0
  Scope1 : Scope  NumInputPorts=4
  cut_theta_2pi : Gain  Gain=(2*pi)/(IncPerTurn*QuadratureFactor)
  cut_theta_2pi1 : Gain  Gain=(2*pi)/(IncPerTurn*QuadratureFactor)
  n_aus_theta_v4 : Subsystem
  rpm : Outport  VectorParamsAs1DForOutWhenUnconnected=off
  theta_mech : Outport  Port=2  VectorParamsAs1DForOutWhenUnconnected=off
  theta_elec : Outport  Port=3  VectorParamsAs1DForOutWhenUnconnected=off
  direction : Outport  Port=4  VectorParamsAs1DForOutWhenUnconnected=off
  wires:
  I/1 -> Counter3/2
  Counter3/1 -> Product/1, cut_theta_2pi/1, Scope1/1
  n_aus_theta_v4/1(n) -> rpm/1
  Logical Operator1/1 -> Scope1/4, Counter3/1
  cut_theta_2pi/1 -> Scope1/2, n_aus_theta_v4/1(theta), theta_mech/1
  Product/1 -> cut_theta_2pi1/1
  poles/1 -> Product/2
  cut_theta_2pi1/1 -> CutTheta_0_2PI/1(In1)
  CutTheta_0_2PI/1(Out1) -> theta_elec/1
  Edge Detector2/1 -> Logical Operator3/1
  Logical Operator4/1 -> Logical Operator3/2
  Logical Operator3/1 -> S-R Flip-Flop1/1
  Edge Detector3/1 -> Logical Operator5/1
  Logical Operator6/1 -> Logical Operator5/2
  Logical Operator5/1 -> S-R Flip-Flop1/2
  S-R Flip-Flop1/1 -> Add/1
  S-R Flip-Flop1/2 -> Add/2
  A/1 -> Logical Operator6/1, Edge Detector2/1, Logical Operator1/1
  B/1 -> Edge Detector3/1, Logical Operator4/1, Logical Operator1/2
  Add/1 -> direction/1

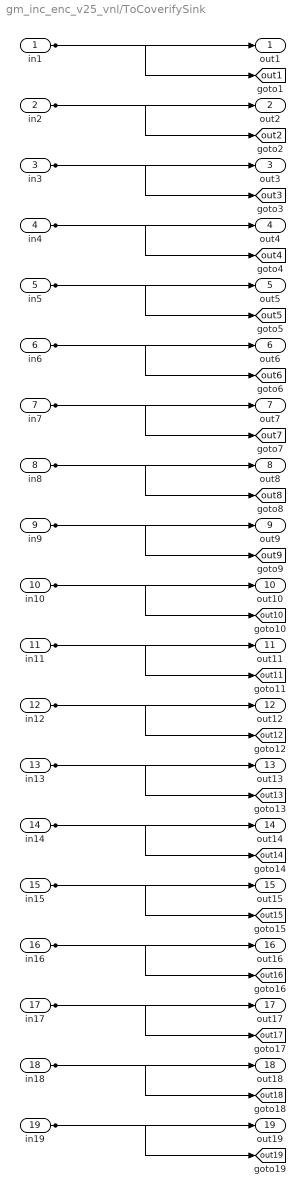
== system gm_inc_enc_v25_vnl/ToCoverifySink ==
  in1 : Inport
  in2 : Inport  Port=2
  in3 : Inport  Port=3
  in4 : Inport  Port=4
  in5 : Inport  Port=5
  in6 : Inport  Port=6
  in7 : Inport  Port=7
  in8 : Inport  Port=8
  in9 : Inport  Port=9
  in10 : Inport  Port=10
  in11 : Inport  Port=11
  in12 : Inport  Port=12
  in13 : Inport  Port=13
  in14 : Inport  Port=14
  in15 : Inport  Port=15
  in16 : Inport  Port=16
  in17 : Inport  Port=17
  in18 : Inport  Port=18
  in19 : Inport  Port=19
  out1 : Outport
  out2 : Outport  Port=2
  out3 : Outport  Port=3
  out4 : Outport  Port=4
  out5 : Outport  Port=5
  out6 : Outport  Port=6
  out7 : Outport  Port=7
  out8 : Outport  Port=8
  out9 : Outport  Port=9
  out10 : Outport  Port=10
  out11 : Outport  Port=11
  out12 : Outport  Port=12
  out13 : Outport  Port=13
  out14 : Outport  Port=14
  out15 : Outport  Port=15
  out16 : Outport  Port=16
  out17 : Outport  Port=17
  out18 : Outport  Port=18
  out19 : Outport  Port=19
  tag scope: out10=global, out11=global, out12=global, out13=global, out14=global, out15=global, out16=global, out17=global, out18=global, out19=global, out1=global, out2=global, out3=global, out4=global, out5=global, out6=global, out7=global, out8=global, out9=global
  wires:
  in1/1 -> out1/1, [out1]
  in2/1 -> out2/1, [out2]
  in3/1 -> out3/1, [out3]
  in4/1 -> out4/1, [out4]
  in5/1 -> out5/1, [out5]
  in6/1 -> out6/1, [out6]
  in7/1 -> out7/1, [out7]
  in8/1 -> out8/1, [out8]
  in9/1 -> out9/1, [out9]
  in10/1 -> out10/1, [out10]
  in11/1 -> out11/1, [out11]
  in12/1 -> out12/1, [out12]
  in13/1 -> out13/1, [out13]
  in14/1 -> out14/1, [out14]
  in15/1 -> out15/1, [out15]
  in16/1 -> out16/1, [out16]
  in17/1 -> out17/1, [out17]
  in18/1 -> out18/1, [out18]
  in19/1 -> out19/1, [out19]

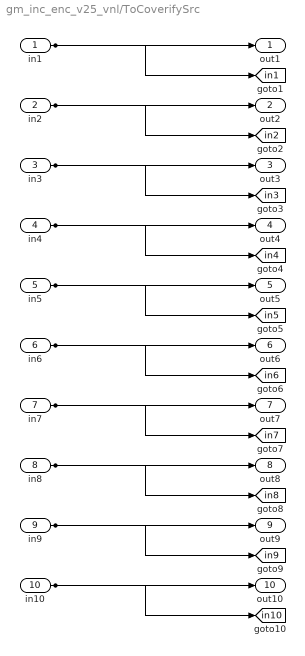
== system gm_inc_enc_v25_vnl/ToCoverifySrc ==
  in1 : Inport
  in2 : Inport  Port=2
  in3 : Inport  Port=3
  in4 : Inport  Port=4
  in5 : Inport  Port=5
  in6 : Inport  Port=6
  in7 : Inport  Port=7
  in8 : Inport  Port=8
  in9 : Inport  Port=9
  in10 : Inport  Port=10
  out1 : Outport
  out2 : Outport  Port=2
  out3 : Outport  Port=3
  out4 : Outport  Port=4
  out5 : Outport  Port=5
  out6 : Outport  Port=6
  out7 : Outport  Port=7
  out8 : Outport  Port=8
  out9 : Outport  Port=9
  out10 : Outport  Port=10
  tag scope: in10=global, in1=global, in2=global, in3=global, in4=global, in5=global, in6=global, in7=global, in8=global, in9=global
  wires:
  in1/1 -> out1/1, [in1]
  in2/1 -> out2/1, [in2]
  in3/1 -> out3/1, [in3]
  in4/1 -> out4/1, [in4]
  in5/1 -> out5/1, [in5]
  in6/1 -> out6/1, [in6]
  in7/1 -> out7/1, [in7]
  in8/1 -> out8/1, [in8]
  in9/1 -> out9/1, [in9]
  in10/1 -> out10/1, [in10]

== system gm_inc_enc_v25_vnl/n_aus_theta ==
  count : Inport
  T : Inport  Port=2
  1/rps->1/omega : Gain  Gain=1/(2*pi)  OutDataTypeStr=double
  Add : Sum  Inputs=+-
  Add1 : Sum
  Constant : Constant  Value=0  OutDataTypeStr=double  SampleTime=-1
  Constant1 : Constant  Value=0  OutDataTypeStr=double  SampleTime=-1
  Constant2 : Constant  Value=0  OutDataTypeStr=double  SampleTime=-1
  Divide1 : Product  Inputs=/
  ProtectOverflow_T_count : Switch  Threshold=50  SaturateOnIntegerOverflow=off  InputSameDT=off
  ProtectOverflow_rps : Switch  Threshold=50  OutDataTypeStr=double  SaturateOnIntegerOverflow=off  InputSameDT=off
  Scope1 : Scope  NumInputPorts=4
  Scope2 : Scope  NumInputPorts=4
  T_count : Delay  DelayLength=1
  T_count_switch : Switch  Criteria=u2 ~= 0  SaturateOnIntegerOverflow=off  InputSameDT=off
  count_old : Delay  DelayLength=1
  count_old_switch : Switch  Criteria=u2 ~= 0  SaturateOnIntegerOverflow=off  InputSameDT=off
  speed_old : Delay  DelayLength=1
  speed_old_switch : Switch  Criteria=u2 ~= 0  SaturateOnIntegerOverflow=off  InputSameDT=off
  rpm : Outport  VectorParamsAs1DForOutWhenUnconnected=off
  wires:
  count_old_switch/1 -> count_old/1
  count_old/1 -> count_old_switch/3, Add/2
  Constant/1 -> T_count_switch/1
  Add/1 -> speed_old_switch/2, count_old_switch/2, Scope1/1, T_count_switch/2
  Constant1/1 -> ProtectOverflow_T_count/1
  ProtectOverflow_rps/1 -> 1/rps->1/omega/1, Scope2/1
  Constant2/1 -> ProtectOverflow_rps/1
  speed_old_switch/1 -> ProtectOverflow_rps/3, Scope2/3, speed_old/1
  speed_old/1 -> speed_old_switch/3
  T/1 -> Scope2/4, Add1/1
  ProtectOverflow_T_count/1 -> T_count/1
  T_count/1 -> Scope1/4, Add1/2
  Add1/1 -> Scope2/2, speed_old_switch/1, T_count_switch/3
  count/1 -> Add/1, count_old_switch/1
  T_count_switch/1 -> ProtectOverflow_rps/2, Scope1/2, ProtectOverflow_T_count/2, ProtectOverflow_T_count/3
  1/rps->1/omega/1 -> Divide1/1
  Divide1/1 -> rpm/1

== system gm_inc_enc_v25_vnl/Compare/Assert_OverSamplFactor ==
  cosim : Inport
  dut : Inport  Port=2
  AssertEq : Assertion  StopWhenAssertionFail=off
  Compare To Zero : simulink/Logic and Bit Operations/Compare To Zero  relop===  OutDataTypeStr=boolean
  Relational Operator : RelationalOperator  Operator===  OutDataTypeStr=boolean  InputSameDT=off
  compare: OverSamplFactor : Scope  NumInputPorts=3
  wires:
  Compare To Zero/1 -> compare: OverSamplFactor/3  "err"
  Relational Operator/1 -> Compare To Zero/1, AssertEq/1
  cosim/1 -> compare: OverSamplFactor/1, Relational Operator/1  "cosim"
  dut/1 -> compare: OverSamplFactor/2, Relational Operator/2  "dut ref"

== system gm_inc_enc_v25_vnl/Compare/Assert_count ==
  cosim : Inport
  dut : Inport  Port=2
  AssertEq : Assertion  StopWhenAssertionFail=off
  Compare To Zero : simulink/Logic and Bit Operations/Compare To Zero  relop===  OutDataTypeStr=boolean
  Relational Operator : RelationalOperator  Operator===  OutDataTypeStr=boolean  InputSameDT=off
  compare: count : Scope  NumInputPorts=3
  wires:
  Compare To Zero/1 -> compare: count/3  "err"
  Relational Operator/1 -> Compare To Zero/1, AssertEq/1
  cosim/1 -> compare: count/1, Relational Operator/1  "cosim"
  dut/1 -> compare: count/2, Relational Operator/2  "dut ref"

== system gm_inc_enc_v25_vnl/Compare/Assert_countPerPeriod_AXI4 ==
  cosim : Inport
  dut : Inport  Port=2
  AssertEq : Assertion  StopWhenAssertionFail=off
  Compare To Zero : simulink/Logic and Bit Operations/Compare To Zero  relop===  OutDataTypeStr=boolean
  Relational Operator : RelationalOperator  Operator===  OutDataTypeStr=boolean  InputSameDT=off
  compare: countPerPeriod_AXI4 : Scope  NumInputPorts=3
  wires:
  Compare To Zero/1 -> compare: countPerPeriod_AXI4/3  "err"
  Relational Operator/1 -> Compare To Zero/1, AssertEq/1
  cosim/1 -> compare: countPerPeriod_AXI4/1, Relational Operator/1  "cosim"
  dut/1 -> compare: countPerPeriod_AXI4/2, Relational Operator/2  "dut ref"

== system gm_inc_enc_v25_vnl/Compare/Assert_direction_AXI4 ==
  cosim : Inport
  dut : Inport  Port=2
  AssertEq : Assertion  StopWhenAssertionFail=off
  Compare To Zero : simulink/Logic and Bit Operations/Compare To Zero  relop===  OutDataTypeStr=boolean
  Relational Operator : RelationalOperator  Operator===  OutDataTypeStr=boolean  InputSameDT=off
  compare: direction_AXI4 : Scope  NumInputPorts=3
  wires:
  Compare To Zero/1 -> compare: direction_AXI4/3  "err"
  Relational Operator/1 -> Compare To Zero/1, AssertEq/1
  cosim/1 -> compare: direction_AXI4/1, Relational Operator/1  "cosim"
  dut/1 -> compare: direction_AXI4/2, Relational Operator/2  "dut ref"

== system gm_inc_enc_v25_vnl/Compare/Assert_edge ==
  cosim : Inport
  dut : Inport  Port=2
  AssertEq : Assertion  StopWhenAssertionFail=off
  Compare To Zero : simulink/Logic and Bit Operations/Compare To Zero  relop===  OutDataTypeStr=boolean
  Relational Operator : RelationalOperator  Operator===  OutDataTypeStr=boolean  InputSameDT=off
  compare: edge : Scope  NumInputPorts=3
  wires:
  Compare To Zero/1 -> compare: edge/3  "err"
  Relational Operator/1 -> Compare To Zero/1, AssertEq/1
  cosim/1 -> compare: edge/1, Relational Operator/1  "cosim"
  dut/1 -> compare: edge/2, Relational Operator/2  "dut ref"

== system gm_inc_enc_v25_vnl/Compare/Assert_new_measurement ==
  cosim : Inport
  dut : Inport  Port=2
  AssertEq : Assertion  StopWhenAssertionFail=off
  Compare To Zero : simulink/Logic and Bit Operations/Compare To Zero  relop===  OutDataTypeStr=boolean
  Relational Operator : RelationalOperator  Operator===  OutDataTypeStr=boolean  InputSameDT=off
  compare: new_measurement : Scope  NumInputPorts=3
  wires:
  Compare To Zero/1 -> compare: new_measurement/3  "err"
  Relational Operator/1 -> Compare To Zero/1, AssertEq/1
  cosim/1 -> compare: new_measurement/1, Relational Operator/1  "cosim"
  dut/1 -> compare: new_measurement/2, Relational Operator/2  "dut ref"

== system gm_inc_enc_v25_vnl/Compare/Assert_omega ==
  cosim : Inport
  dut : Inport  Port=2
  AssertEq : Assertion  StopWhenAssertionFail=off
  Compare To Zero : simulink/Logic and Bit Operations/Compare To Zero  relop===  OutDataTypeStr=boolean
  Relational Operator : RelationalOperator  Operator===  OutDataTypeStr=boolean  InputSameDT=off
  compare: omega : Scope  NumInputPorts=3
  wires:
  Compare To Zero/1 -> compare: omega/3  "err"
  Relational Operator/1 -> Compare To Zero/1, AssertEq/1
  cosim/1 -> compare: omega/1, Relational Operator/1  "cosim"
  dut/1 -> compare: omega/2, Relational Operator/2  "dut ref"

== system gm_inc_enc_v25_vnl/Compare/Assert_omegaA ==
  cosim : Inport
  dut : Inport  Port=2
  AssertEq : Assertion  StopWhenAssertionFail=off
  Compare To Zero : simulink/Logic and Bit Operations/Compare To Zero  relop===  OutDataTypeStr=boolean
  Relational Operator : RelationalOperator  Operator===  OutDataTypeStr=boolean  InputSameDT=off
  compare: omegaA : Scope  NumInputPorts=3
  wires:
  Compare To Zero/1 -> compare: omegaA/3  "err"
  Relational Operator/1 -> Compare To Zero/1, AssertEq/1
  cosim/1 -> compare: omegaA/1, Relational Operator/1  "cosim"
  dut/1 -> compare: omegaA/2, Relational Operator/2  "dut ref"

== system gm_inc_enc_v25_vnl/Compare/Assert_omegaB ==
  cosim : Inport
  dut : Inport  Port=2
  AssertEq : Assertion  StopWhenAssertionFail=off
  Compare To Zero : simulink/Logic and Bit Operations/Compare To Zero  relop===  OutDataTypeStr=boolean
  Relational Operator : RelationalOperator  Operator===  OutDataTypeStr=boolean  InputSameDT=off
  compare: omegaB : Scope  NumInputPorts=3
  wires:
  Compare To Zero/1 -> compare: omegaB/3  "err"
  Relational Operator/1 -> Compare To Zero/1, AssertEq/1
  cosim/1 -> compare: omegaB/1, Relational Operator/1  "cosim"
  dut/1 -> compare: omegaB/2, Relational Operator/2  "dut ref"

== system gm_inc_enc_v25_vnl/Compare/Assert_omegaNOTA ==
  cosim : Inport
  dut : Inport  Port=2
  AssertEq : Assertion  StopWhenAssertionFail=off
  Compare To Zero : simulink/Logic and Bit Operations/Compare To Zero  relop===  OutDataTypeStr=boolean
  Relational Operator : RelationalOperator  Operator===  OutDataTypeStr=boolean  InputSameDT=off
  compare: omegaNOTA : Scope  NumInputPorts=3
  wires:
  Compare To Zero/1 -> compare: omegaNOTA/3  "err"
  Relational Operator/1 -> Compare To Zero/1, AssertEq/1
  cosim/1 -> compare: omegaNOTA/1, Relational Operator/1  "cosim"
  dut/1 -> compare: omegaNOTA/2, Relational Operator/2  "dut ref"

== system gm_inc_enc_v25_vnl/Compare/Assert_omegaNOTB ==
  cosim : Inport
  dut : Inport  Port=2
  AssertEq : Assertion  StopWhenAssertionFail=off
  Compare To Zero : simulink/Logic and Bit Operations/Compare To Zero  relop===  OutDataTypeStr=boolean
  Relational Operator : RelationalOperator  Operator===  OutDataTypeStr=boolean  InputSameDT=off
  compare: omegaNOTB : Scope  NumInputPorts=3
  wires:
  Compare To Zero/1 -> compare: omegaNOTB/3  "err"
  Relational Operator/1 -> Compare To Zero/1, AssertEq/1
  cosim/1 -> compare: omegaNOTB/1, Relational Operator/1  "cosim"
  dut/1 -> compare: omegaNOTB/2, Relational Operator/2  "dut ref"

== system gm_inc_enc_v25_vnl/Compare/Assert_omega_AXI4 ==
  cosim : Inport
  dut : Inport  Port=2
  AssertEq : Assertion  StopWhenAssertionFail=off
  Compare To Zero : simulink/Logic and Bit Operations/Compare To Zero  relop===  OutDataTypeStr=boolean
  Relational Operator : RelationalOperator  Operator===  OutDataTypeStr=boolean  InputSameDT=off
  compare: omega_AXI4 : Scope  NumInputPorts=3
  wires:
  Compare To Zero/1 -> compare: omega_AXI4/3  "err"
  Relational Operator/1 -> Compare To Zero/1, AssertEq/1
  cosim/1 -> compare: omega_AXI4/1, Relational Operator/1  "cosim"
  dut/1 -> compare: omega_AXI4/2, Relational Operator/2  "dut ref"

== system gm_inc_enc_v25_vnl/Compare/Assert_omega_MA_N4 ==
  cosim : Inport
  dut : Inport  Port=2
  AssertEq : Assertion  StopWhenAssertionFail=off
  Compare To Zero : simulink/Logic and Bit Operations/Compare To Zero  relop===  OutDataTypeStr=boolean
  Relational Operator : RelationalOperator  Operator===  OutDataTypeStr=boolean  InputSameDT=off
  compare: omega_MA_N4 : Scope  NumInputPorts=3
  wires:
  Compare To Zero/1 -> compare: omega_MA_N4/3  "err"
  Relational Operator/1 -> Compare To Zero/1, AssertEq/1
  cosim/1 -> compare: omega_MA_N4/1, Relational Operator/1  "cosim"
  dut/1 -> compare: omega_MA_N4/2, Relational Operator/2  "dut ref"

== system gm_inc_enc_v25_vnl/Compare/Assert_omega_MA_N4_AXI ==
  cosim : Inport
  dut : Inport  Port=2
  AssertEq : Assertion  StopWhenAssertionFail=off
  Compare To Zero : simulink/Logic and Bit Operations/Compare To Zero  relop===  OutDataTypeStr=boolean
  Relational Operator : RelationalOperator  Operator===  OutDataTypeStr=boolean  InputSameDT=off
  compare: omega_MA_N4_AXI : Scope  NumInputPorts=3
  wires:
  Compare To Zero/1 -> compare: omega_MA_N4_AXI/3  "err"
  Relational Operator/1 -> Compare To Zero/1, AssertEq/1
  cosim/1 -> compare: omega_MA_N4_AXI/1, Relational Operator/1  "cosim"
  dut/1 -> compare: omega_MA_N4_AXI/2, Relational Operator/2  "dut ref"

== system gm_inc_enc_v25_vnl/Compare/Assert_position ==
  cosim : Inport
  dut : Inport  Port=2
  AssertEq : Assertion  StopWhenAssertionFail=off
  Compare To Zero : simulink/Logic and Bit Operations/Compare To Zero  relop===  OutDataTypeStr=boolean
  Relational Operator : RelationalOperator  Operator===  OutDataTypeStr=boolean  InputSameDT=off
  compare: position : Scope  NumInputPorts=3
  wires:
  Compare To Zero/1 -> compare: position/3  "err"
  Relational Operator/1 -> Compare To Zero/1, AssertEq/1
  cosim/1 -> compare: position/1, Relational Operator/1  "cosim"
  dut/1 -> compare: position/2, Relational Operator/2  "dut ref"

== system gm_inc_enc_v25_vnl/Compare/Assert_position_AXI4 ==
  cosim : Inport
  dut : Inport  Port=2
  AssertEq : Assertion  StopWhenAssertionFail=off
  Compare To Zero : simulink/Logic and Bit Operations/Compare To Zero  relop===  OutDataTypeStr=boolean
  Relational Operator : RelationalOperator  Operator===  OutDataTypeStr=boolean  InputSameDT=off
  compare: position_AXI4 : Scope  NumInputPorts=3
  wires:
  Compare To Zero/1 -> compare: position_AXI4/3  "err"
  Relational Operator/1 -> Compare To Zero/1, AssertEq/1
  cosim/1 -> compare: position_AXI4/1, Relational Operator/1  "cosim"
  dut/1 -> compare: position_AXI4/2, Relational Operator/2  "dut ref"
